simulink model "spectrum_fft_hdlcoder"  (R2020a)
settings: Solver=FixedStepAuto  StartTime=0.0  StopTime=inf  RelTol=1e-3
InitFcn:
  | spectrum_fft_setup;
values from neighbouring files (symbols this model uses):
  BufferLength = 2048    [spectrum_fft_setup.m]
  f = 256e6    (= 256000000)    [spectrum_fft_setup.m]
  fc_rx = 128e6    (= 128000000)    [spectrum_fft_setup.m]
  fc_tx = 64e6    (= 64000000)    [spectrum_fft_setup.m]
  fs = 1.024e9    (= 1024000000)    [spectrum_fft_setup.m]
  SymbolRate = 1e6    (= 1000000)    [spectrum_fft_setup.m]
undefined symbols (not defined in the file or in its folder): designMultirateFIR, F_CICI, F_RRC, FFT, firhalfband, lib_fft
libraries: dspmlti4 x6, simulink x4, hdlsllib x4, dspfdesign x4, dsparch4 x2, dspsrcs4 x2, commfilt2 x2, dsphdlxfrm x1, commrandsrc3 x1, commdigbbndpm3 x1
settings Model: DataTypeOverride=Off  SimulationMode=accelerator  Creator=rgb11127  LastModifiedBy=david
settings DataIOCC: SaveOutput=off  SaveTime=off
settings OptimizationCC: BlockReduction=off  ConditionallyExecuteInputs=off  DefaultParameterBehavior=Inlined
settings DebuggingCC: AlgebraicLoopMsg=error  SingleTaskRateTransMsg=error
settings HardwareCC: ProdBitPerPointer=32  ProdBitPerSizeT=32  ProdBitPerPtrDiffT=32  ProdLargestAtomicFloat=None  ProdIntDivRoundTo=Undefined  ProdEndianess=Unspecified  ProdWordSize=32  ProdHWDeviceType=ASIC/FPGA->ASIC/FPGA  TargetBitPerPointer=64  TargetBitPerSizeT=64  TargetBitPerPtrDiffT=64  TargetLongLongMode=on  TargetIntDivRoundTo=Zero  TargetEndianess=LittleEndian  TargetWordSize=64  TargetHWDeviceType=Custom Processor->MATLAB Host Computer  ProdEqTarget=off
settings SFSimCC: CustomCodeUndefinedFunction=UseInterfaceOnly

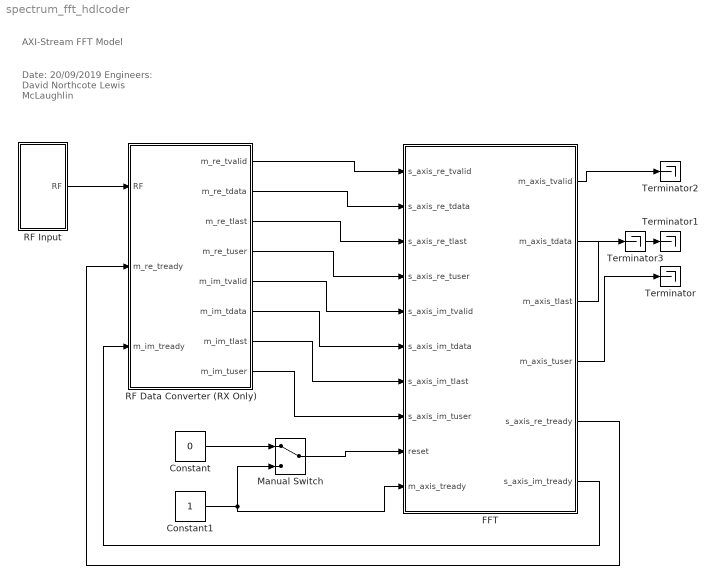
== system spectrum_fft_hdlcoder ==
  note: Date:		20/09/2019
      | Engineers:	David Northcote
      | 			Lewis McLaughlin
  note: AXI-Stream FFT Model
  Constant : Constant  Value=0  OutDataTypeStr=boolean  SampleTime=1/f
  Constant1 : Constant  OutDataTypeStr=boolean  SampleTime=1/f
  FFT : Subsystem  AncestorBlock=lib_fft/FFT  TreatAsAtomicUnit=on
  Manual Switch : ManualSwitch
  RF Data Converter (RX Only) : Subsystem
  RF Input : Subsystem  Variant=on  VariantControlMode=Label  VariantControl=Variant1  LabelModeActiveChoice=Variant1
  Terminator{,1..3} (4 alike) : Terminator
  wires:
  RF Data Converter (RX Only)/1(m_re_tvalid) -> FFT/1(s_axis_re_tvalid)
  RF Data Converter (RX Only)/2(m_re_tdata) -> FFT/2(s_axis_re_tdata)
  RF Data Converter (RX Only)/6(m_im_tdata) -> FFT/6(s_axis_im_tdata)
  FFT/4(m_axis_tuser) -> Terminator/1
  FFT/3(m_axis_tlast) -> Terminator1/1
  FFT/1(m_axis_tvalid) -> Terminator2/1
  RF Data Converter (RX Only)/3(m_re_tlast) -> FFT/3(s_axis_re_tlast)
  RF Data Converter (RX Only)/4(m_re_tuser) -> FFT/4(s_axis_re_tuser)
  RF Data Converter (RX Only)/5(m_im_tvalid) -> FFT/5(s_axis_im_tvalid)
  RF Data Converter (RX Only)/7(m_im_tlast) -> FFT/7(s_axis_im_tlast)
  RF Data Converter (RX Only)/8(m_im_tuser) -> FFT/8(s_axis_im_tuser)
  FFT/5(s_axis_re_tready) -> RF Data Converter (RX Only)/2(m_re_tready)
  FFT/6(s_axis_im_tready) -> RF Data Converter (RX Only)/3(m_im_tready)
  Manual Switch/1 -> FFT/9(reset)
  Constant/1 -> Manual Switch/1
  Constant1/1 -> Manual Switch/2, FFT/10(m_axis_tready)
  RF Input/1(RF) -> RF Data Converter (RX Only)/1(RF)
  FFT/2(m_axis_tdata) -> Terminator3/1

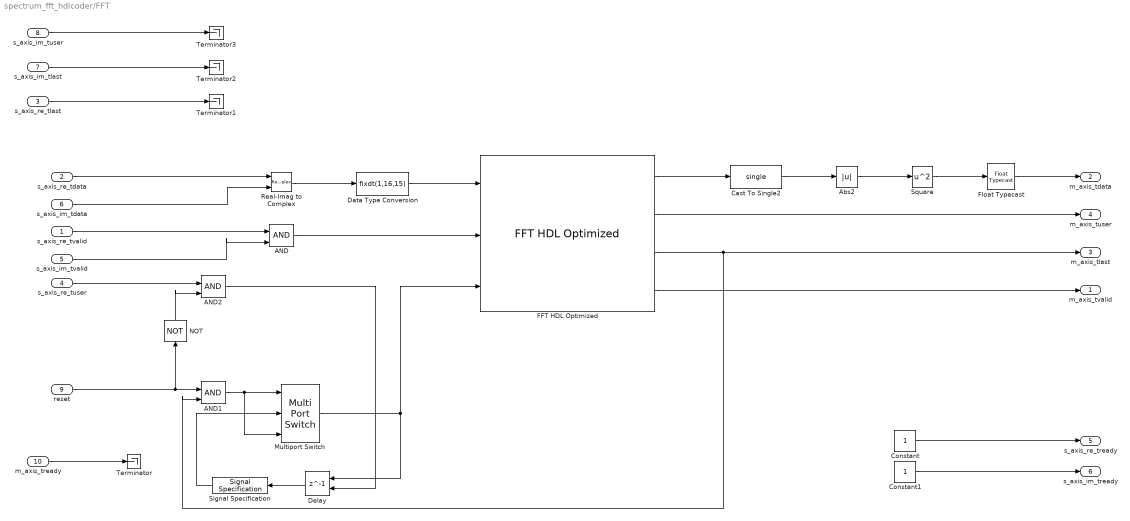
== system spectrum_fft_hdlcoder/FFT ==
  s_axis_re_tvalid : Inport
  s_axis_re_tdata : Inport  Port=2
  s_axis_re_tlast : Inport  Port=3
  s_axis_re_tuser : Inport  Port=4
  s_axis_im_tvalid : Inport  Port=5
  s_axis_im_tdata : Inport  Port=6
  s_axis_im_tlast : Inport  Port=7
  s_axis_im_tuser : Inport  Port=8
  reset : Inport  Port=9
  m_axis_tready : Inport  Port=10
  AND : Logic  IconShape=distinctive  AllPortsSameDT=off  OutDataTypeStr=boolean
  AND1 : Logic  IconShape=distinctive  AllPortsSameDT=off  OutDataTypeStr=boolean
  AND2 : Logic  IconShape=distinctive  AllPortsSameDT=off  OutDataTypeStr=boolean
  Abs2 : Abs
  Cast To Single2 : DataTypeConversion  OutDataTypeStr=single
  Constant : Constant  OutDataTypeStr=boolean  SampleTime=1/f
  Constant1 : Constant  OutDataTypeStr=boolean  SampleTime=1/f
  Data Type Conversion : DataTypeConversion  OutDataTypeStr=fixdt(1,16,15)  ConvertRealWorld=Stored Integer (SI)
  Delay : Delay  DelayLength=1  ExternalReset=Level
      settings: InputPortMap=u0,r5
  FFT HDL Optimized : dsphdlxfrm/FFT HDL Optimized  FFTLength=2048  Architecture=Streaming Radix 2^2  ComplexMultiplication=Use 4 multipliers and 2 adders  BitReversedOutput=off  BitReversedInput=off  Normalize=off  SimulateUsing=Code generation  RoundingMethod=Floor  ResetInputPort=on  StartOutputPort=on  EndOutputPort=on
      settings: SourceProductBaseCode=DS
  Float Typecast : FloatTypecast
  Multiport Switch : MultiPortSwitch  DataPortOrder=Zero-based contiguous  Inputs=2  zeroidx=on
  NOT : Logic  Operator=NOT  IconShape=distinctive  AllPortsSameDT=off  OutDataTypeStr=boolean
  Real-Imag to Complex : RealImagToComplex
  Signal Specification : SignalSpecification  OutDataTypeStr=boolean
  Square : Math  Operator=square  SaturateOnIntegerOverflow=on
  Terminator{,1..3} (4 alike) : Terminator
  m_axis_tvalid : Outport  VectorParamsAs1DForOutWhenUnconnected=off
  m_axis_tdata : Outport  Port=2  VectorParamsAs1DForOutWhenUnconnected=off
  m_axis_tlast : Outport  Port=3  VectorParamsAs1DForOutWhenUnconnected=off
  m_axis_tuser : Outport  Port=4  VectorParamsAs1DForOutWhenUnconnected=off
  s_axis_re_tready : Outport  Port=5  VectorParamsAs1DForOutWhenUnconnected=off
  s_axis_im_tready : Outport  Port=6  VectorParamsAs1DForOutWhenUnconnected=off
  wires:
  FFT HDL Optimized/1 -> Cast To Single2/1
  Real-Imag to Complex/1 -> Data Type Conversion/1
  AND/1 -> FFT HDL Optimized/2
  s_axis_re_tlast/1 -> Terminator1/1
  s_axis_im_tlast/1 -> Terminator2/1
  s_axis_im_tuser/1 -> Terminator3/1
  Constant/1 -> s_axis_re_tready/1
  AND1/1 -> Multiport Switch/3, Multiport Switch/1
  Multiport Switch/1 -> FFT HDL Optimized/3, Delay/1
  NOT/1 -> AND2/2
  AND2/1 -> Delay/2
  Delay/1 -> Signal Specification/1
  Signal Specification/1 -> Multiport Switch/2
  m_axis_tready/1 -> Terminator/1
  Data Type Conversion/1 -> FFT HDL Optimized/1
  s_axis_re_tdata/1 -> Real-Imag to Complex/1
  s_axis_im_tdata/1 -> Real-Imag to Complex/2
  s_axis_re_tvalid/1 -> AND/1
  s_axis_im_tvalid/1 -> AND/2
  s_axis_re_tuser/1 -> AND2/1
  reset/1 -> NOT/1, AND1/1
  FFT HDL Optimized/2 -> m_axis_tuser/1
  FFT HDL Optimized/3 -> m_axis_tlast/1, AND1/2
  FFT HDL Optimized/4 -> m_axis_tvalid/1
  Cast To Single2/1 -> Abs2/1
  Abs2/1 -> Square/1
  Square/1 -> Float Typecast/1
  Constant1/1 -> s_axis_im_tready/1
  Float Typecast/1 -> m_axis_tdata/1

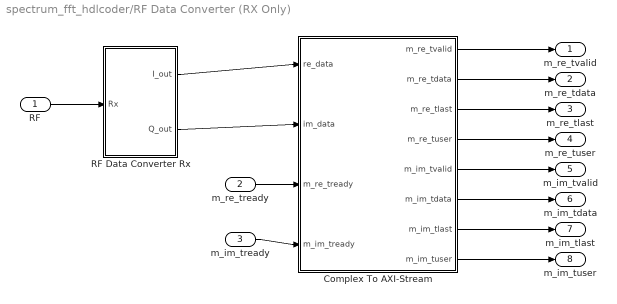
== system spectrum_fft_hdlcoder/RF Data Converter (RX Only) ==
  RF : Inport
  m_re_tready : Inport  Port=2
  m_im_tready : Inport  Port=3
  Complex To AXI-Stream : Subsystem
  RF Data Converter Rx : Subsystem
  m_re_tvalid : Outport  VectorParamsAs1DForOutWhenUnconnected=off
  m_re_tdata : Outport  Port=2  VectorParamsAs1DForOutWhenUnconnected=off
  m_re_tlast : Outport  Port=3  VectorParamsAs1DForOutWhenUnconnected=off
  m_re_tuser : Outport  Port=4  VectorParamsAs1DForOutWhenUnconnected=off
  m_im_tvalid : Outport  Port=5  VectorParamsAs1DForOutWhenUnconnected=off
  m_im_tdata : Outport  Port=6  VectorParamsAs1DForOutWhenUnconnected=off
  m_im_tlast : Outport  Port=7  VectorParamsAs1DForOutWhenUnconnected=off
  m_im_tuser : Outport  Port=8  VectorParamsAs1DForOutWhenUnconnected=off
  wires:
  Complex To AXI-Stream/4(m_re_tuser) -> m_re_tuser/1
  RF Data Converter Rx/1(I_out) -> Complex To AXI-Stream/1(re_data)
  m_re_tready/1 -> Complex To AXI-Stream/3(m_re_tready)
  RF Data Converter Rx/2(Q_out) -> Complex To AXI-Stream/2(im_data)
  m_im_tready/1 -> Complex To AXI-Stream/4(m_im_tready)
  Complex To AXI-Stream/2(m_re_tdata) -> m_re_tdata/1
  RF/1 -> RF Data Converter Rx/1(Rx)
  Complex To AXI-Stream/8(m_im_tuser) -> m_im_tuser/1
  Complex To AXI-Stream/6(m_im_tdata) -> m_im_tdata/1
  Complex To AXI-Stream/5(m_im_tvalid) -> m_im_tvalid/1
  Complex To AXI-Stream/1(m_re_tvalid) -> m_re_tvalid/1
  Complex To AXI-Stream/3(m_re_tlast) -> m_re_tlast/1
  Complex To AXI-Stream/7(m_im_tlast) -> m_im_tlast/1

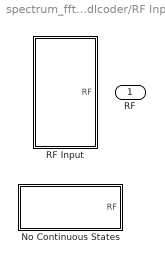
== system spectrum_fft_hdlcoder/RF Input ==
  No Continuous States : Subsystem  VariantControl=Choice
  RF Input : Subsystem  VariantControl=Variant1
  RF : Outport  VectorParamsAs1DForOutWhenUnconnected=off

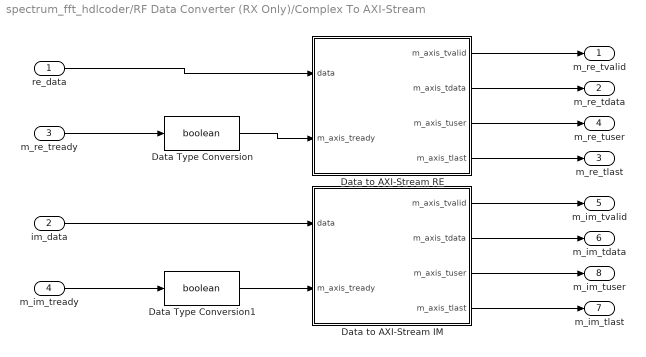
== system spectrum_fft_hdlcoder/RF Data Converter (RX Only)/Complex To AXI-Stream ==
  re_data : Inport
  im_data : Inport  Port=2
  m_re_tready : Inport  Port=3
  m_im_tready : Inport  Port=4
  Data Type Conversion : DataTypeConversion  OutDataTypeStr=boolean
  Data Type Conversion1 : DataTypeConversion  OutDataTypeStr=boolean
  Data to AXI-Stream IM : Subsystem
  Data to AXI-Stream RE : Subsystem
  m_re_tvalid : Outport  VectorParamsAs1DForOutWhenUnconnected=off
  m_re_tdata : Outport  Port=2  VectorParamsAs1DForOutWhenUnconnected=off
  m_re_tlast : Outport  Port=3  VectorParamsAs1DForOutWhenUnconnected=off
  m_re_tuser : Outport  Port=4  VectorParamsAs1DForOutWhenUnconnected=off
  m_im_tvalid : Outport  Port=5  VectorParamsAs1DForOutWhenUnconnected=off
  m_im_tdata : Outport  Port=6  VectorParamsAs1DForOutWhenUnconnected=off
  m_im_tlast : Outport  Port=7  VectorParamsAs1DForOutWhenUnconnected=off
  m_im_tuser : Outport  Port=8  VectorParamsAs1DForOutWhenUnconnected=off
  wires:
  Data to AXI-Stream RE/3(m_axis_tuser) -> m_re_tuser/1
  im_data/1 -> Data to AXI-Stream IM/1(data)
  Data to AXI-Stream IM/3(m_axis_tuser) -> m_im_tuser/1
  Data to AXI-Stream IM/2(m_axis_tdata) -> m_im_tdata/1
  m_re_tready/1 -> Data Type Conversion/1
  Data to AXI-Stream RE/2(m_axis_tdata) -> m_re_tdata/1
  m_im_tready/1 -> Data Type Conversion1/1
  re_data/1 -> Data to AXI-Stream RE/1(data)
  Data Type Conversion/1 -> Data to AXI-Stream RE/2(m_axis_tready)
  Data Type Conversion1/1 -> Data to AXI-Stream IM/2(m_axis_tready)
  Data to AXI-Stream RE/1(m_axis_tvalid) -> m_re_tvalid/1
  Data to AXI-Stream IM/1(m_axis_tvalid) -> m_im_tvalid/1
  Data to AXI-Stream RE/4(m_axis_tlast) -> m_re_tlast/1
  Data to AXI-Stream IM/4(m_axis_tlast) -> m_im_tlast/1

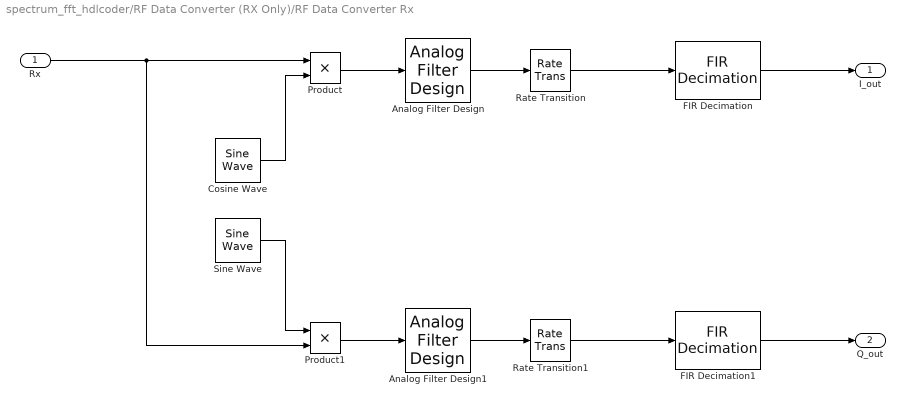
== system spectrum_fft_hdlcoder/RF Data Converter (RX Only)/RF Data Converter Rx ==
  Rx : Inport
  Analog Filter Design : dsparch4/Analog Filter Design  method=Butterworth  filttype=Lowpass  N=8  Wlo=2*pi*128e6  Whi=80  Rp=2  Rs=40
  Analog Filter Design1 : dsparch4/Analog Filter Design  method=Butterworth  filttype=Lowpass  N=8  Wlo=2*pi*128e6  Whi=80  Rp=2  Rs=40
  Cosine Wave : dspsrcs4/Sine Wave  Amplitude=1  Frequency=fc_rx  Phase=pi/2  SampleMode=Continuous  OutComplex=Real  CompMethod=Trigonometric fcn  TableSize=Speed  SampleTime=0  SamplesPerFrame=1  ResetState=Restart at time zero  OutputFrames=off  dataType=double  wordLen=16  udDataType=sfix(16)  fracBitsMode=Best precision  numFracBits=15  OutDataTypeStr=double  LastOutDataTypeStr=double
  FIR Decimation : dspmlti4/FIR Decimation  FilterSource=Auto  h=designMultirateFIR(1,2)  D=4  filtStruct=Direct form  FilterObject=FDECIM  framing=Enforce single-rate processing  inputOffset=0  outputBufInitCond=0  roundingMode=Floor  overflowMode=off  firstCoeffDataTypeStr=Inherit: Same word length as input  firstCoeffMin=[]  firstCoeffMax=[]  firstCoeffLastDataTypeStr=Inherit: Same word length as input  outputDataTypeStr=Inherit: Same as accumulator  outputMin=[]  outputMax=[]  outputLastDataTypeStr=Inherit: Same as accumulator
  FIR Decimation1 : dspmlti4/FIR Decimation  FilterSource=Auto  h=designMultirateFIR(1,2)  D=4  filtStruct=Direct form  FilterObject=FDECIM  framing=Enforce single-rate processing  inputOffset=0  outputBufInitCond=0  roundingMode=Floor  overflowMode=off  firstCoeffDataTypeStr=Inherit: Same word length as input  firstCoeffMin=[]  firstCoeffMax=[]  firstCoeffLastDataTypeStr=Inherit: Same word length as input  outputDataTypeStr=Inherit: Same as accumulator  outputMin=[]  outputMax=[]  outputLastDataTypeStr=Inherit: Same as accumulator
  Product : Product
  Product1 : Product
  Rate Transition : RateTransition  OutPortSampleTime=1/fs
  Rate Transition1 : RateTransition  OutPortSampleTime=1/fs
  Sine Wave : dspsrcs4/Sine Wave  Amplitude=1  Frequency=fc_rx  Phase=pi  SampleMode=Continuous  OutComplex=Real  CompMethod=Trigonometric fcn  TableSize=Speed  SampleTime=1/f  SamplesPerFrame=1  ResetState=Restart at time zero  OutputFrames=off  dataType=double  wordLen=16  udDataType=sfix(16)  fracBitsMode=Best precision  numFracBits=15  OutDataTypeStr=double  LastOutDataTypeStr=double
  I_out : Outport  VectorParamsAs1DForOutWhenUnconnected=off
  Q_out : Outport  Port=2  VectorParamsAs1DForOutWhenUnconnected=off
  wires:
  FIR Decimation1/1 -> Q_out/1
  Sine Wave/1 -> Product1/1
  Cosine Wave/1 -> Product/2
  Rx/1 -> Product/1, Product1/2
  Rate Transition1/1 -> FIR Decimation1/1
  FIR Decimation/1 -> I_out/1
  Rate Transition/1 -> FIR Decimation/1
  Product/1 -> Analog Filter Design/1
  Product1/1 -> Analog Filter Design1/1
  Analog Filter Design/1 -> Rate Transition/1
  Analog Filter Design1/1 -> Rate Transition1/1

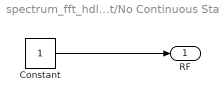
== system spectrum_fft_hdlcoder/RF Input/No Continuous States ==
  Constant : Constant  OutDataTypeStr=double  SampleTime=1/(f*4)
  RF : Outport  VectorParamsAs1DForOutWhenUnconnected=off
  wires:
  Constant/1 -> RF/1

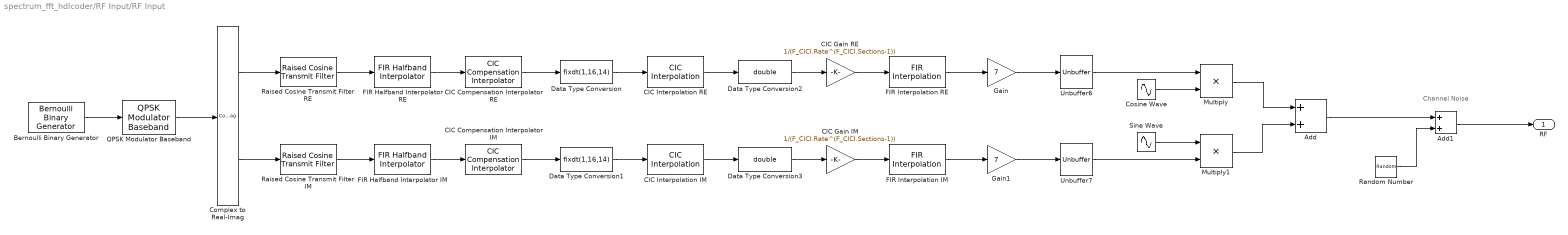
== system spectrum_fft_hdlcoder/RF Input/RF Input ==
  note: Channel Noise
  Add : Sum
  Add1 : Sum
  Bernoulli Binary Generator : commrandsrc3/Bernoulli Binary Generator  ProbabilityOfZero=0.5  SeedSource=Parameter  Seed=0  SampleTime=1/(SymbolRate*2)  SamplesPerFrame=2  OutputDataType=double  SimulateUsing=Interpreted execution
  CIC Interpolation IM : dspmlti4/CIC Interpolation  filtFrom=Dialog parameters  filtobj=CICINTERP  ftype=Interpolator  R=F_CICI.Rate  M=F_CICI.DifferentialDelay  N=F_CICI.Sections  filterInternals=Full precision  BPS=[16 16 16 16]  FLPS=0  outputWordLength=32  outputFracLength=0  launchFVT=off  InputProcessing=Columns as channels (frame based)  framing=Enforce single-rate processing  OutputFrames=off
      settings: SourceProductBaseCode=DS
  CIC Interpolation RE : dspmlti4/CIC Interpolation  filtFrom=Dialog parameters  filtobj=CICINTERP  ftype=Interpolator  R=F_CICI.Rate  M=F_CICI.DifferentialDelay  N=F_CICI.Sections  filterInternals=Full precision  BPS=[16 16 16 16]  FLPS=0  outputWordLength=32  outputFracLength=0  launchFVT=off  InputProcessing=Columns as channels (frame based)  framing=Enforce single-rate processing  OutputFrames=off
      settings: SourceProductBaseCode=DS
  CIC Compensation Interpolator IM : dspfdesign/CIC Compensation Interpolator  CICRateChangeFactor=F_CICI.Rate  CICNumSections=F_CICI.Sections  CICDifferentialDelay=F_CICI.DifferentialDelay  InterpolationFactor=F_CICC.Rate  DesignForMinimumOrder=on  FilterOrder=12  PassbandFrequency=F_CICC.Passband  StopbandFrequency=F_CICC.Stopband  PassbandRipple=F_CICC.Ripple  StopbandAttenuation=F_CICC.StopbandAttenuation  InheritSampleRate=off  SampleRate=F_CICC.SampleRate  SimulateUsing=Code generation  roundingMode=Floor  coeffsDataTypeStr=fixdt(1,16)
      settings: SourceProductBaseCode=DS
  CIC Compensation Interpolator RE : dspfdesign/CIC Compensation Interpolator  CICRateChangeFactor=F_CICI.Rate  CICNumSections=F_CICI.Sections  CICDifferentialDelay=F_CICI.DifferentialDelay  InterpolationFactor=F_CICC.Rate  DesignForMinimumOrder=on  FilterOrder=12  PassbandFrequency=F_CICC.Passband  StopbandFrequency=F_CICC.Stopband  PassbandRipple=F_CICC.Ripple  StopbandAttenuation=F_CICC.StopbandAttenuation  InheritSampleRate=off  SampleRate=F_CICC.SampleRate  SimulateUsing=Code generation  roundingMode=Floor  coeffsDataTypeStr=fixdt(1,16)
      settings: SourceProductBaseCode=DS
  CIC Gain IM : Gain  Gain=1/(F_CICI.Rate^(F_CICI.Sections-1))
  CIC Gain RE : Gain  Gain=1/(F_CICI.Rate^(F_CICI.Sections-1))
  Complex to Real-Imag : ComplexToRealImag
  Cosine Wave : Sin  Frequency=2*pi*fc_tx  Phase=pi/2  SampleTime=0
  Data Type Conversion : DataTypeConversion  OutDataTypeStr=fixdt(1,16,14)
  Data Type Conversion1 : DataTypeConversion  OutDataTypeStr=fixdt(1,16,14)
  Data Type Conversion2 : DataTypeConversion  OutDataTypeStr=double
  Data Type Conversion3 : DataTypeConversion  OutDataTypeStr=double
  FIR Interpolation IM : dspmlti4/FIR Interpolation  FilterSource=Auto  PrivateCoeffs=0  h=designMultirateFIR(3,1)  L=8  FilterObject=FINTERP  InputProcessing=Columns as channels (frame based)  framing=Enforce single-rate processing  outputBufInitCond=0  roundingMode=Floor  overflowMode=off  firstCoeffDataTypeStr=Inherit: Same word length as input  firstCoeffMin=[]  firstCoeffMax=[]  firstCoeffLastDataTypeStr=Inherit: Same word length as input  outputDataTypeStr=Inherit: Same as accumulator  outputMin=[]  outputMax=[]  outputLastDataTypeStr=Inherit: Same as accumulator
  FIR Interpolation RE : dspmlti4/FIR Interpolation  FilterSource=Auto  PrivateCoeffs=0  h=designMultirateFIR(3,1)  L=8  FilterObject=FINTERP  InputProcessing=Columns as channels (frame based)  framing=Enforce single-rate processing  outputBufInitCond=0  roundingMode=Floor  overflowMode=off  firstCoeffDataTypeStr=Inherit: Same word length as input  firstCoeffMin=[]  firstCoeffMax=[]  firstCoeffLastDataTypeStr=Inherit: Same word length as input  outputDataTypeStr=Inherit: Same as accumulator  outputMin=[]  outputMax=[]  outputLastDataTypeStr=Inherit: Same as accumulator
  FIR Halfband Interpolator IM : dspfdesign/FIR Halfband Interpolator  Specification=Transition width and stopband attenuation  FilterOrder=52  TransitionWidth=F_HB.TransitionWidth  StopbandAttenuation=F_HB.StopbandAttenuation  Numerator=2*firhalfband( 'minorder', 0.407, 1e-4 )  FilterBankInputPort=off  InheritSampleRate=off  SampleRate=F_HB.SampleRate  SimulateUsing=Code generation  roundingMode=Floor  coeffsDataTypeStr=fixdt(1,16)
      settings: SourceProductBaseCode=DS
  FIR Halfband Interpolator RE : dspfdesign/FIR Halfband Interpolator  Specification=Transition width and stopband attenuation  FilterOrder=52  TransitionWidth=F_HB.TransitionWidth  StopbandAttenuation=F_HB.StopbandAttenuation  Numerator=2*firhalfband( 'minorder', 0.407, 1e-4 )  FilterBankInputPort=off  InheritSampleRate=off  SampleRate=F_HB.SampleRate  SimulateUsing=Code generation  roundingMode=Floor  coeffsDataTypeStr=fixdt(1,16)
      settings: SourceProductBaseCode=DS
  Gain : Gain  Gain=7
  Gain1 : Gain  Gain=7
  Multiply : Product
  Multiply1 : Product
  QPSK Modulator Baseband : commdigbbndpm3/QPSK Modulator Baseband  InType=Bit  Enc=Gray  Ph=pi/4  outDtype=double  outWordLen=16  outUDDataType=sfix(16)  outFracLenMode=Best precision  outFracLen=15  outDataTypeStr=double  outLastDataTypeStr=double
  Raised Cosine Transmit Filter IM : commfilt2/Raised Cosine Transmit Filter  filtType=Square root  R=F_RRC.RollOff  filtSpan=F_RRC.FilterSpan  N=F_RRC.Rate  filterGain=F_RRC.LinearGain  InputProcessing=Columns as channels (frame based)  RateOptions=Allow multirate processing  framing=Mute  checkCoeff=off  variableName=rcTxFilt1  checkGain=Normalized  sampMode=Mute  saveAsFlag=0  currentFiltSpan=10  D=(10)/2  launchFVT=on  roundingMode=Floor  overflowMode=off  coeffDataTypeStr=Inherit: Same word length as input  coeffMin=[]  coeffMax=[]  coeffLastDataTypeStr=Inherit: Same word length as input  outputDataTypeStr=Inherit: Same as accumulator  outputMin=[]  outputMax=[]  outputLastDataTypeStr=Inherit: Same as accumulator
  Raised Cosine Transmit Filter RE : commfilt2/Raised Cosine Transmit Filter  filtType=Square root  R=F_RRC.RollOff  filtSpan=F_RRC.FilterSpan  N=F_RRC.Rate  filterGain=F_RRC.LinearGain  InputProcessing=Columns as channels (frame based)  RateOptions=Allow multirate processing  framing=Mute  checkCoeff=off  variableName=rcTxFilt  checkGain=Normalized  sampMode=Mute  saveAsFlag=0  currentFiltSpan=10  D=(10)/2  launchFVT=on  roundingMode=Floor  overflowMode=off  coeffDataTypeStr=Inherit: Same word length as input  coeffMin=[]  coeffMax=[]  coeffLastDataTypeStr=Inherit: Same word length as input  outputDataTypeStr=Inherit: Same as accumulator  outputMin=[]  outputMax=[]  outputLastDataTypeStr=Inherit: Same as accumulator
  Random Number : RandomNumber  Variance=0.05
  Sine Wave : Sin  Frequency=2*pi*fc_tx  SampleTime=0
  Unbuffer6 : Unbuffer
  Unbuffer7 : Unbuffer
  RF : Outport  VectorParamsAs1DForOutWhenUnconnected=off
  wires:
  Bernoulli Binary Generator/1 -> QPSK Modulator Baseband/1
  Complex to Real-Imag/1 -> Raised Cosine Transmit Filter RE/1
  QPSK Modulator Baseband/1 -> Complex to Real-Imag/1
  Complex to Real-Imag/2 -> Raised Cosine Transmit Filter IM/1
  Raised Cosine Transmit Filter RE/1 -> FIR Halfband Interpolator RE/1
  Raised Cosine Transmit Filter IM/1 -> FIR Halfband Interpolator IM/1
  FIR Halfband Interpolator RE/1 -> CIC Compensation Interpolator RE/1
  FIR Halfband Interpolator IM/1 -> CIC Compensation Interpolator IM/1
  CIC Compensation Interpolator RE/1 -> Data Type Conversion/1
  CIC Compensation Interpolator IM/1 -> Data Type Conversion1/1
  CIC Interpolation RE/1 -> Data Type Conversion2/1
  Data Type Conversion/1 -> CIC Interpolation RE/1
  Data Type Conversion1/1 -> CIC Interpolation IM/1
  Data Type Conversion2/1 -> CIC Gain RE/1
  Data Type Conversion3/1 -> CIC Gain IM/1
  CIC Interpolation IM/1 -> Data Type Conversion3/1
  CIC Gain RE/1 -> FIR Interpolation RE/1
  CIC Gain IM/1 -> FIR Interpolation IM/1
  Multiply/1 -> Add/1
  Multiply1/1 -> Add/2
  FIR Interpolation RE/1 -> Gain/1
  Cosine Wave/1 -> Multiply/2
  Sine Wave/1 -> Multiply1/1
  FIR Interpolation IM/1 -> Gain1/1
  Unbuffer6/1 -> Multiply/1
  Unbuffer7/1 -> Multiply1/2
  Gain/1 -> Unbuffer6/1
  Gain1/1 -> Unbuffer7/1
  Add/1 -> Add1/1
  Add1/1 -> RF/1
  Random Number/1 -> Add1/2

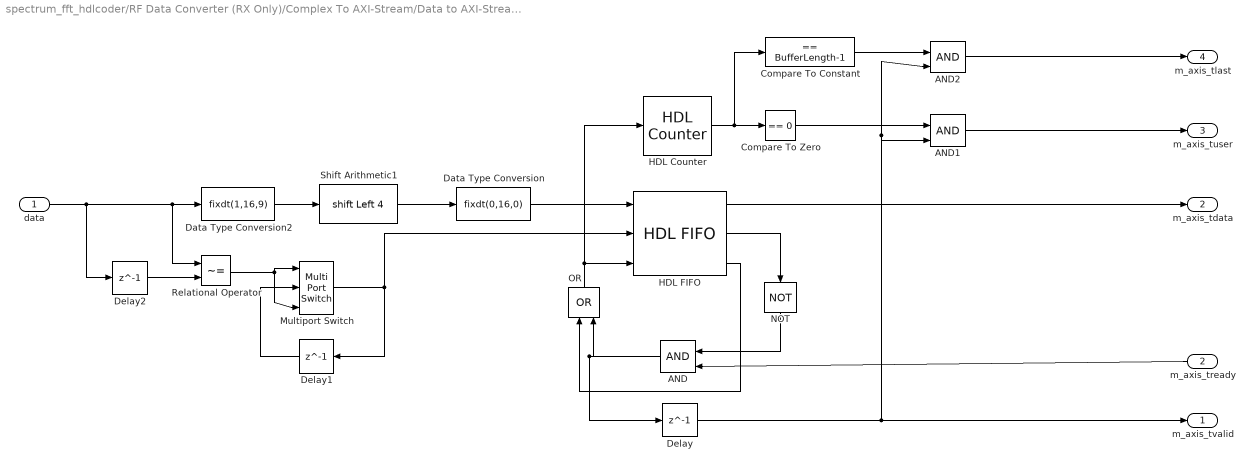
== system spectrum_fft_hdlcoder/RF Data Converter (RX Only)/Complex To AXI-Stream/Data to AXI-Stream IM ==
  data : Inport
  m_axis_tready : Inport  Port=2
  AND : Logic  IconShape=distinctive  AllPortsSameDT=off  OutDataTypeStr=boolean
  AND1 : Logic  IconShape=distinctive  AllPortsSameDT=off  OutDataTypeStr=boolean
  AND2 : Logic  IconShape=distinctive  AllPortsSameDT=off  OutDataTypeStr=boolean
  Compare To Constant : simulink/Logic and Bit Operations/Compare To Constant  relop===  const=BufferLength-1  OutDataTypeStr=boolean
  Compare To Zero : simulink/Logic and Bit Operations/Compare To Zero  relop===  OutDataTypeStr=boolean
  Data Type Conversion : DataTypeConversion  OutDataTypeStr=fixdt(0,16,0)  ConvertRealWorld=Stored Integer (SI)
  Data Type Conversion2 : DataTypeConversion  OutDataTypeStr=fixdt(1,16,9)
  Delay : Delay  DelayLength=1
  Delay1 : Delay  DelayLength=1
  Delay2 : Delay  DelayLength=1
  HDL Counter : hdlsllib/Sources/HDL Counter  CountType=Count limited  CountInit=0  CountStep=1  CountMax=BufferLength-1  CountFromType=Initial value  CountFrom=0  CountResetPort=off  CountLoadPort=off  CountEnbPort=on  CountDirPort=off  CountDataType=Unsigned  CountWordLen=32  CountFracLen=0  CountSampTime=1
  HDL FIFO : hdlsllib/HDL RAMs/HDL FIFO  fifo_size=256  mode=Classic  ratio=1  push_msg=Error  pop_msg=Error  show_empty=on  show_full=on  show_num=off  LabelModeActiveChoice_Mode=Classic
      settings: SourceProductBaseCode=SL
  Multiport Switch : MultiPortSwitch  DataPortOrder=Zero-based contiguous  Inputs=2  zeroidx=on
  NOT : Logic  Operator=NOT  IconShape=distinctive  AllPortsSameDT=off  OutDataTypeStr=boolean
  OR : Logic  Operator=OR  IconShape=distinctive  AllPortsSameDT=off  OutDataTypeStr=boolean
  Relational Operator : RelationalOperator  Operator=~=  OutDataTypeStr=boolean  RndMeth=Simplest
  Shift Arithmetic1 : ArithShift  BitShiftNumber=4  BitShiftDirection=Left
  m_axis_tvalid : Outport  VectorParamsAs1DForOutWhenUnconnected=off
  m_axis_tdata : Outport  Port=2  VectorParamsAs1DForOutWhenUnconnected=off
  m_axis_tuser : Outport  Port=3  VectorParamsAs1DForOutWhenUnconnected=off
  m_axis_tlast : Outport  Port=4  VectorParamsAs1DForOutWhenUnconnected=off
  wires:
  AND2/1 -> m_axis_tlast/1
  Compare To Constant/1 -> AND2/1
  Data Type Conversion/1 -> HDL FIFO/1
  Shift Arithmetic1/1 -> Data Type Conversion/1
  Data Type Conversion2/1 -> Shift Arithmetic1/1
  OR/1 -> HDL Counter/1, HDL FIFO/3
  HDL FIFO/3 -> OR/1
  AND/1 -> OR/2, Delay/1
  Delay2/1 -> Relational Operator/2
  Relational Operator/1 -> Multiport Switch/1, Multiport Switch/3
  Delay1/1 -> Multiport Switch/2
  Multiport Switch/1 -> Delay1/1, HDL FIFO/2
  data/1 -> Data Type Conversion2/1, Relational Operator/1, Delay2/1
  m_axis_tready/1 -> AND/2
  NOT/1 -> AND/1
  Delay/1 -> m_axis_tvalid/1, AND1/2, AND2/2
  HDL FIFO/2 -> NOT/1
  HDL Counter/1 -> Compare To Zero/1, Compare To Constant/1
  Compare To Zero/1 -> AND1/1
  AND1/1 -> m_axis_tuser/1
  HDL FIFO/1 -> m_axis_tdata/1

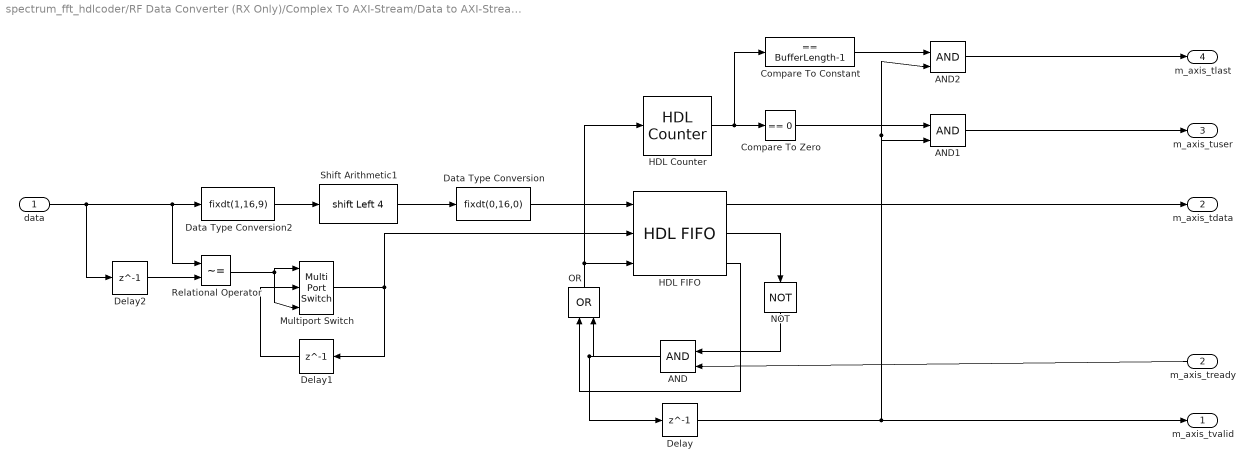
== system spectrum_fft_hdlcoder/RF Data Converter (RX Only)/Complex To AXI-Stream/Data to AXI-Stream RE ==
  data : Inport
  m_axis_tready : Inport  Port=2
  AND : Logic  IconShape=distinctive  AllPortsSameDT=off  OutDataTypeStr=boolean
  AND1 : Logic  IconShape=distinctive  AllPortsSameDT=off  OutDataTypeStr=boolean
  AND2 : Logic  IconShape=distinctive  AllPortsSameDT=off  OutDataTypeStr=boolean
  Compare To Constant : simulink/Logic and Bit Operations/Compare To Constant  relop===  const=BufferLength-1  OutDataTypeStr=boolean
  Compare To Zero : simulink/Logic and Bit Operations/Compare To Zero  relop===  OutDataTypeStr=boolean
  Data Type Conversion : DataTypeConversion  OutDataTypeStr=fixdt(0,16,0)  ConvertRealWorld=Stored Integer (SI)
  Data Type Conversion2 : DataTypeConversion  OutDataTypeStr=fixdt(1,16,9)
  Delay : Delay  DelayLength=1
  Delay1 : Delay  DelayLength=1
  Delay2 : Delay  DelayLength=1
  HDL Counter : hdlsllib/Sources/HDL Counter  CountType=Count limited  CountInit=0  CountStep=1  CountMax=BufferLength-1  CountFromType=Initial value  CountFrom=0  CountResetPort=off  CountLoadPort=off  CountEnbPort=on  CountDirPort=off  CountDataType=Unsigned  CountWordLen=32  CountFracLen=0  CountSampTime=1
  HDL FIFO : hdlsllib/HDL RAMs/HDL FIFO  fifo_size=256  mode=Classic  ratio=1  push_msg=Error  pop_msg=Error  show_empty=on  show_full=on  show_num=off  LabelModeActiveChoice_Mode=Classic
      settings: SourceProductBaseCode=SL
  Multiport Switch : MultiPortSwitch  DataPortOrder=Zero-based contiguous  Inputs=2  zeroidx=on
  NOT : Logic  Operator=NOT  IconShape=distinctive  AllPortsSameDT=off  OutDataTypeStr=boolean
  OR : Logic  Operator=OR  IconShape=distinctive  AllPortsSameDT=off  OutDataTypeStr=boolean
  Relational Operator : RelationalOperator  Operator=~=  OutDataTypeStr=boolean  RndMeth=Simplest
  Shift Arithmetic1 : ArithShift  BitShiftNumber=4  BitShiftDirection=Left
  m_axis_tvalid : Outport  VectorParamsAs1DForOutWhenUnconnected=off
  m_axis_tdata : Outport  Port=2  VectorParamsAs1DForOutWhenUnconnected=off
  m_axis_tuser : Outport  Port=3  VectorParamsAs1DForOutWhenUnconnected=off
  m_axis_tlast : Outport  Port=4  VectorParamsAs1DForOutWhenUnconnected=off
  wires:
  HDL FIFO/1 -> m_axis_tdata/1
  AND1/1 -> m_axis_tuser/1
  Compare To Zero/1 -> AND1/1
  HDL Counter/1 -> Compare To Constant/1, Compare To Zero/1
  HDL FIFO/2 -> NOT/1
  Delay/1 -> AND2/2, AND1/2, m_axis_tvalid/1
  NOT/1 -> AND/1
  m_axis_tready/1 -> AND/2
  data/1 -> Delay2/1, Relational Operator/1, Data Type Conversion2/1
  Multiport Switch/1 -> HDL FIFO/2, Delay1/1
  Delay1/1 -> Multiport Switch/2
  Relational Operator/1 -> Multiport Switch/3, Multiport Switch/1
  Delay2/1 -> Relational Operator/2
  AND/1 -> Delay/1, OR/2
  HDL FIFO/3 -> OR/1
  OR/1 -> HDL FIFO/3, HDL Counter/1
  Data Type Conversion2/1 -> Shift Arithmetic1/1
  Shift Arithmetic1/1 -> Data Type Conversion/1
  Data Type Conversion/1 -> HDL FIFO/1
  Compare To Constant/1 -> AND2/1
  AND2/1 -> m_axis_tlast/1
